simulink library "DataLogger"  (R2016b)
settings: Solver=VariableStepAuto  StartTime=0.0  StopTime=10.0  RelTol=1e-3
libraries: DatalogHandler x1, LatchHandler x1, ScopeHandler x1
settings Model: Creator=Nathan  LastModifiedBy=march

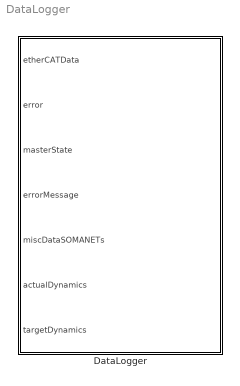
== system DataLogger ==
  DataLogger : Subsystem

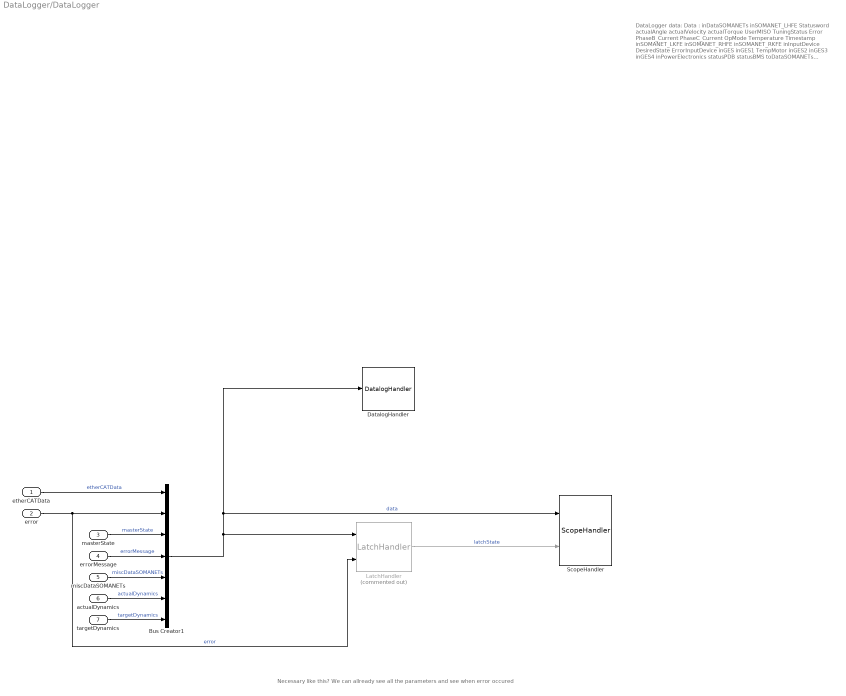
== system DataLogger/DataLogger ==
  note: DataLogger data:
      | Data :
      | inDataSOMANETs
      | inSOMANET_LHFE
      | Statusword
      | actualAngle
      | actualVelocity
      | actualTorque
      | UserMISO
      | TuningStatus
      | Error
      | PhaseB_Current
      | PhaseC_Current
      | OpMode
      | Temperature
      | Timestamp
      | inSOMANET_LKFE
      | inSOMANET_RHFE
      | inSOMANET_RKFE
      | inInputDevice
      | DesiredState
      | ErrorInputDevice
      | inGES
      | inGES1
      | TempMotor
      | inGES2
      | inGES3
      | inGES4
      | inPowerElectronics
      | statusPDB
      | statusBMS
      | toDataSOMANETs
      | toSOMANET_LHFE
      | Controlword
      | OpMode
      | targetAngle
      | targetVelocity
      | targetTorque
      | TuningCommand
      | UserMOSI
      | maxTorque
      | toSOMANET_LKFE
      | toSOMANET_RHFE
      | toSOMANET_RKFE
      | toInputDevice
      | actualStateMARCH
      | Error
      | toPowerElectronics
      | toPDB
      | MasterOP
      | toGES
      | -
      | Error
      | ErrorSOMANETs
      | ErrorSOMANET_LHFE
      | ErrorSOMANET_LKFE
      | ErrorSOMANET_RHFE
      | ErrorSOMANET_RKFE
      | ErrorInputDevice
      | ErrorGES
      | ErrorGES1
      | ErrorGES2
      | ErrorGES3
      | ErrorGES4
      | ErrorPowerElectronics
      | ErrorPDB
      | ErrorBMS
      | GaitPhase
      | actualStateMARCH
      | ConfigSOMANETs
      | AngleOffset
      | PolePairs
      | minPosLimit
      | maxPosLimit
      | maxSpeed
      | maxTorque
      | PositionKp
      | PositionKi
      | PositionKd
      | PositionIntegralLimit
      | VelocityKp
      | VelocityKi
      | VelocityKd
      | VelocityIntegralLimit
      | BreakReleaseStrategy
      | calculatedDynamics
      | LatchState :
      | All data on specific error moment
  note: Necessary like this? We can allready see all the parameters and see when error occured
  etherCATData : Inport  OutDataTypeStr=Bus: EtherCATData  PortDimensions=[1 4]  LockScale=on  BusOutputAsStruct=on
  error : Inport  Port=2  OutDataTypeStr=Bus: DeviceErrors  BusOutputAsStruct=on
  masterState : Inport  Port=3
  errorMessage : Inport  Port=4
  miscDataSOMANETs : Inport  Port=5  OutDataTypeStr=Bus: MiscDataSOMANET  BusOutputAsStruct=on
  actualDynamics : Inport  Port=6
  targetDynamics : Inport  Port=7
  Bus Creator1 : BusCreator  Inputs=7  OutDataTypeStr=Bus: ExoskeletonData  NonVirtualBus=on
  DatalogHandler : DatalogHandler/DatalogHandler
  LatchHandler : LatchHandler/LatchHandler  Commented=on
  ScopeHandler : ScopeHandler/ScopeHandler
  wires:
  targetDynamics/1 -> Bus Creator1/7  "targetDynamics"
  actualDynamics/1 -> Bus Creator1/6  "actualDynamics"
  miscDataSOMANETs/1 -> Bus Creator1/5  "miscDataSOMANETs"
  errorMessage/1 -> Bus Creator1/4  "errorMessage"
  masterState/1 -> Bus Creator1/3  "masterState"
  error/1 -> Bus Creator1/2, LatchHandler/2  "error"
  etherCATData/1 -> Bus Creator1/1  "etherCATData"
  LatchHandler/1 -> ScopeHandler/2  "latchState"
  Bus Creator1/1 -> LatchHandler/1, ScopeHandler/1, DatalogHandler/1  "data"
